simulink model "SingleMerging"  (R2018b)
settings: Solver=VariableStepAuto  StartTime=0.0  StopTime=30  FixedStep=0.1  RelTol=1e-3
PreLoadFcn:
  | init_func
values from neighbouring files (symbols this model uses):
  m = 1650    [CBF_Control.m]    (also in acc.m)
settings Model: Creator=nebneBgnahZ  LastModifiedBy=admin
settings SFSimCC: SimUseLocalCustomCode=off
settings RTWCC: RTWUseLocalCustomCode=off
settings CodeAppCC: StateflowObjectComments=on

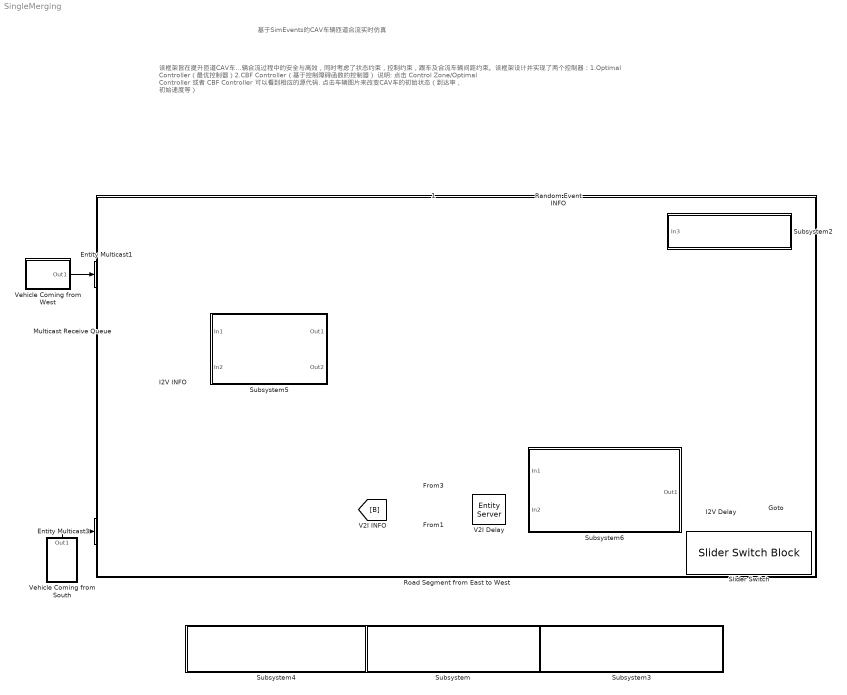
== system SingleMerging ==
  note: 该框架旨在提升匝道CAV车辆合流过程中的安全与高效，同时考虑了状态约束，控制约束，跟车及合流车辆间距约束。该框架设计并实现了两个控制器：1.Optimal Controller（最优控制器）2.CBF Controller（基于控制障碍函数的控制器）
      | 说明:
      | 点击 Control Zone/Optimal Controller 或者 CBF Controller 可以看到相应的源代码.
      | 点击车辆图片来改变CAV车的初始状态（到达率， 初始速度等）
  note: 基于SimEvents的CAV车辆匝道合流实时仿真
  " 1" : Subsystem  mask(Random events){Parameter1=Red Light Violation Warning}
      mask help: Random events do not only refer to vehicle arrival, lane change, and turn, but they also include events that may cause safety issues. Generally, all such random events can be categorized into two classes, depending on whether they are caused by vehicles or by the infrastructure/environment.
      mask TypeOptions Parameter1: Red Light Violation Warning | Curve Speed Warning | Stop Sign Gap Assist | Spot Weather Impact Warning | Reduced Speed/ Work Zone Warning | Pedestrian in Signalized Crosswalk Warning (Transit) | Emergency Electronic Brake Lights (EEBL) | Forward Collision Warning (FCW) | Intersection Movement Assist (IMA) | Left Turn Assist (LTA) | Blind Spot/ Lane Change Warning (BSW/LCW) | Do Not Pass Warning (DNPW) | Vehicle Turning Right in Front of Bus Warning (Transit)
      mask Display:
      | %image('figs/environment.jpg');
      | disp('Random Events')
  Entity Multicast1 : EntityMulticast  InputPortMessageModes=m  MulticastTag=CAV
  Entity Multicast3 : EntityMulticast  InputPortMessageModes=m  MulticastTag=CAV
  I2V Delay : EntityServer  InputPortMessageModes=m  OutputPortMessageModes=m  Capacity=Inf  ServiceTimeValue=0
  Multicast Receive Queue : EntityQueue  OutputPortMessageModes=m  Capacity=100  EntityArrivalSource=Multicast  MulticastTag=CAV
      settings: OutputPortMap=o5
  Road Segment from East to West : Subsystem
      mask Display: image('figs/mergbkg.png');
  Slider Switch : SliderSwitchBlock  WebBlockId=192  LabelPosition=Hide
      settings: Values={{'OC', 'CBF'}, [1 2]}
  Subsystem : Subsystem
      settings: OpenFcn=edit dynamics.m
      mask Display: disp('OC Vehicle Dynamics');
  Subsystem2 : Subsystem
      mask Display: disp('Merging Point')
  Subsystem3 : Subsystem
      settings: OpenFcn=edit fuel_consumption.m
      mask Display: disp('Fuel Consumption Model');
  Subsystem4 : Subsystem
      settings: OpenFcn=edit acc.m
      mask Display: disp('CBF Vehicle Dynamics');
  Subsystem5 : Subsystem
      mask Display:
      | %image('figs/controller.jpg');
      | disp('Control Zone')
  Subsystem6 : Subsystem
      mask Display:
      | %image('figs/coordinator.jpg');
      | disp('Coordinator')
  V2I Delay : EntityServer  InputPortMessageModes=m  OutputPortMessageModes=m  Capacity=Inf  ServiceTimeValue=0.1
  Vehicle Coming from South : Subsystem  mask(Connected Automated Vehicles (CAVs)){modelpopup=Basic model, umin=[], umax=[], vmin=[], vmax=[], length=0, cf=0, cr=0, lf=0, lr=0}
      mask prompts: modelpopup "Vehicle Model Selection"; umin "Maximum Deceleration"; umax "Maximum Acceleration"; vmin "Minimum Speed"; vmax "Maximum Speed"; cf "Front Tire Cornering Stiffness"; cr "Rear Tire Cornering Stiffness"; lf "Distance from CoG to Front Axels"; lr "Distance from CoG to Rear Axels"
      mask help: Vehicles, assumed to be CAVs, should possess the ability to communicate with the controller, the coordinator, and other vehicles in the network. CAVs can differ in driver models, for instance, motion dynamics, control mechanism, and fuel consumption dynamics.
      mask TypeOptions modelpopup: Basic model | Kinematic model | Dynamic model | User-defined
      mask Callback modelpopup:
      | % Get the mask parameter values. This is a cell
      | %   array of character vectors.
      | maskStr = get_param(gcb,'modelpopup');
      | 
      | % The pop-up menu is the first mask parameter.
      | %   Check the value selected in the pop-up
      | if strcmp(maskStr(1),'U')
      | 
      | 
      |     % Set the visibility of both parameters on when
      |     %   User-defined is selected in the pop-up.
      | 
      |     set_param(gcb,'MaskVisibilities',{'on';'on';'on';'on';'on';'on';'on';'on';'on';'on';}),
      | 
      | elseif strcmp(maskStr(1),'B')
      | 
      |     % Turn off the visibility of the Value field
      |     %   when User-defined is not selected.
      | 
      |     set_param(gcb,'MaskVisibilities',{'on';'on';'on';'on';'on';'off';'off';'off';'off';'off';}),
      | 
      |     % Set the character vector in the Values field equal to the
      |     % character vector selected in the Gain pop-up menu.
      | 
      |     %maskStr{2}=maskStr{1};
      | 
      | 
      | elseif strcmp(maskStr(1),'K')
      | 
      |     set_param(gcb,'MaskVisibilities',{'on';'on';'on';'on';'on';'on';'off';'off';'off';'off';}),
      | 
      | else
      | 
      |     set_param(gcb,'MaskVisibilities',{'on';'on';'on';'on';'on';'off';'on';'on';'on';'on';}),
      | 
      | end
      mask Display: image('figs/CAV2.png');
  Vehicle Coming from West : Subsystem  mask(Connected Automated Vehicles (CAVs)){modelpopup=Basic model, umin=[], umax=[], vmin=[], vmax=[], length=0, cf=0, cr=0, lf=0, lr=0}
      mask prompts: modelpopup "Vehicle Model Selection"; umin "Maximum Deceleration"; umax "Maximum Acceleration"; vmin "Minimum Speed"; vmax "Maximum Speed"; cf "Front Tire Cornering Stiffness"; cr "Rear Tire Cornering Stiffness"; lf "Distance from CoG to Front Axels"; lr "Distance from CoG to Rear Axels"
      mask help: Vehicles, assumed to be CAVs, should possess the ability to communicate with the controller, the coordinator, and other vehicles in the network. CAVs can differ in driver models, for instance, motion dynamics, control mechanism, and fuel consumption dynamics.
      mask TypeOptions modelpopup: Basic model | Kinematic model | Dynamic model | User-defined
      mask Callback modelpopup:
      | % Get the mask parameter values. This is a cell
      | %   array of character vectors.
      | maskStr = get_param(gcb,'modelpopup');
      | 
      | % The pop-up menu is the first mask parameter.
      | %   Check the value selected in the pop-up
      | if strcmp(maskStr(1),'U')
      | 
      | 
      |     % Set the visibility of both parameters on when
      |     %   User-defined is selected in the pop-up.
      | 
      |     set_param(gcb,'MaskVisibilities',{'on';'on';'on';'on';'on';'on';'on';'on';'on';'on';}),
      | 
      | elseif strcmp(maskStr(1),'B')
      | 
      |     % Turn off the visibility of the Value field
      |     %   when User-defined is not selected.
      | 
      |     set_param(gcb,'MaskVisibilities',{'on';'on';'on';'on';'on';'off';'off';'off';'off';'off';}),
      | 
      |     % Set the character vector in the Values field equal to the
      |     % character vector selected in the Gain pop-up menu.
      | 
      |     %maskStr{2}=maskStr{1};
      | 
      | 
      | elseif strcmp(maskStr(1),'K')
      | 
      |     set_param(gcb,'MaskVisibilities',{'on';'on';'on';'on';'on';'on';'off';'off';'off';'off';}),
      | 
      | else
      | 
      |     set_param(gcb,'MaskVisibilities',{'on';'on';'on';'on';'on';'off';'on';'on';'on';'on';}),
      | 
      | end
      mask Display: image('figs/CAV.png');
  wires:
  Vehicle Coming from South/1(Out1) -> Entity Multicast3/1
  Vehicle Coming from West/1(Out1) -> Entity Multicast1/1
  I2V Delay/1 -> [A]
  [B] -> V2I Delay/1
  " 1"/1(Out1) -> [C]
  Multicast Receive Queue/1 -> Subsystem5/1(In1)
  [A] -> Subsystem5/2(In2)
  Subsystem5/2(Out2) -> [B]
  [C] -> Subsystem6/1(In1)
  Subsystem6/1(Out1) -> I2V Delay/1
  Subsystem5/1(Out1) -> Subsystem2/1(In3)
  V2I Delay/1 -> Subsystem6/2(In2)

== system SingleMerging/ 1 ==
  Random Event : EntityGenerator  OutputPortMessageModes=m  TimeSource=MATLAB action  IntergenerationTimeAction=dt = 1000;  GenerateEntityAtSimulationStart=off  AttributeName=entity  AttributeInitialValue=0  EntityType=Bus object  EntityTypeName=INFO  EntityPriority=100
  Out1 : Outport
  wires:
  Random Event/1 -> Out1/1

== system SingleMerging/Road Segment from East to West ==

== system SingleMerging/Subsystem ==

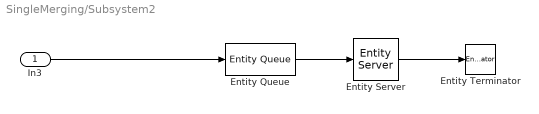
== system SingleMerging/Subsystem2 ==
  In3 : Inport
  Entity Queue : EntityQueue  InputPortMessageModes=m  OutputPortMessageModes=m
      settings: OutputPortMap=o5
  Entity Server : EntityServer  InputPortMessageModes=m  OutputPortMessageModes=m  Capacity=Inf  ServiceTimeSource=MATLAB action  ServiceTimeAction=dt = 30 / entity.FinalSpeed;
  Entity Terminator : EntityTerminator  InputPortMessageModes=m
  wires:
  Entity Queue/1 -> Entity Server/1
  In3/1 -> Entity Queue/1
  Entity Server/1 -> Entity Terminator/1

== system SingleMerging/Subsystem3 ==

== system SingleMerging/Subsystem4 ==

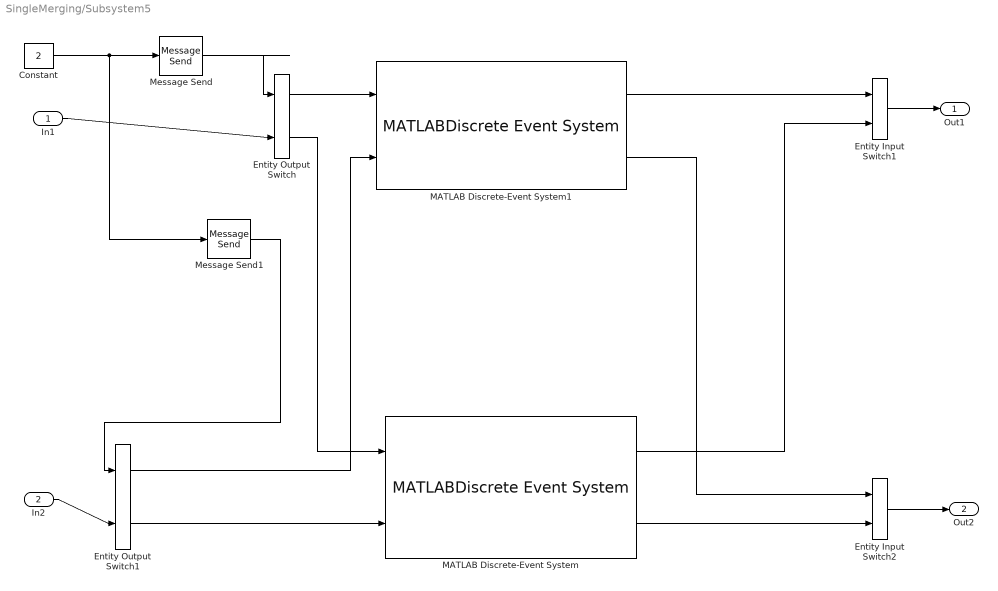
== system SingleMerging/Subsystem5 ==
  In1 : Inport
  In2 : Inport  Port=2
  Constant : Constant  Value=2  SampleTime=-1
  Entity Input Switch1 : EntityInputSwitch  InputPortMessageModes=m,m  OutputPortMessageModes=m  SwitchingCriterion=From control port
  Entity Input Switch2 : EntityInputSwitch  InputPortMessageModes=m,m  OutputPortMessageModes=m  SwitchingCriterion=From control port
  Entity Output Switch : EntityOutputSwitch  InputPortMessageModes=m,m  OutputPortMessageModes=m,m  SwitchingCriterion=From control port  SwitchAttributeName=Attribute1
      settings: InputPortMap=u0,u1
  Entity Output Switch1 : EntityOutputSwitch  InputPortMessageModes=m,m  OutputPortMessageModes=m,m  SwitchingCriterion=From control port  SwitchAttributeName=Attribute1
      settings: InputPortMap=u0,u1
  MATLAB Discrete-Event System : MATLABDiscreteEventSystem  InputPortMessageModes=m,m  OutputPortMessageModes=m,m  System=CBFController  capacity=100  Length=400  step=0.1  Vd=30  Vmax=30  Vmin=0  Umax=0.4  Umin=0.6  SimulateUsing=Interpreted execution
      mask Type: CBFController
      mask Display:
      | disp('CBF Controller');
      | port_label('input',1,'IN');
      | port_label('input',2,'INFO');
      | port_label('output',1,'OUT');
      | port_label('output',2,'INFO');
  MATLAB Discrete-Event System1 : MATLABDiscreteEventSystem  Description=Coordinator  InputPortMessageModes=m,m  OutputPortMessageModes=m,m  System=Controller  capacity=100  step=0.1  L=400  SimulateUsing=Interpreted execution
      mask Type: Controller
      mask Display:
      | disp('OPTIMAL CONTROLLER');
      | port_label('input',1,'IN');
      | port_label('input',2,'INFO');
      | port_label('output',1,'OUT');
      | port_label('output',2,'INFO');
  Message Send : MessageSend  OutputPortMessageModes=m
      settings: InputPortMap=u1
  Message Send1 : MessageSend  OutputPortMessageModes=m
      settings: InputPortMap=u1
  Out1 : Outport
  Out2 : Outport  Port=2
  wires:
  Message Send/1 -> Entity Output Switch/1
  Entity Output Switch1/2 -> MATLAB Discrete-Event System/2
  Entity Output Switch1/1 -> MATLAB Discrete-Event System1/2
  Entity Output Switch/1 -> MATLAB Discrete-Event System1/1
  MATLAB Discrete-Event System/1 -> Entity Input Switch1/2
  MATLAB Discrete-Event System/2 -> Entity Input Switch2/2
  In2/1 -> Entity Output Switch1/2
  Entity Input Switch1/1 -> Out1/1
  Entity Input Switch2/1 -> Out2/1
  Entity Output Switch/2 -> MATLAB Discrete-Event System/1
  MATLAB Discrete-Event System1/2 -> Entity Input Switch2/1
  In1/1 -> Entity Output Switch/2
  Constant/1 -> Message Send/1, Message Send1/1
  MATLAB Discrete-Event System1/1 -> Entity Input Switch1/1
  Message Send1/1 -> Entity Output Switch1/1

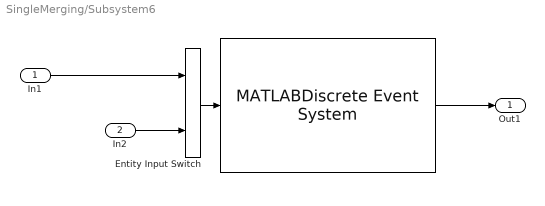
== system SingleMerging/Subsystem6 ==
  In1 : Inport
  In2 : Inport  Port=2
  " " : MATLABDiscreteEventSystem  InputPortMessageModes=m  OutputPortMessageModes=m  System=Coordinator  capacity=100  SimulateUsing=Interpreted execution
      mask Type: Coordinator
      mask Display:
      | disp('COORDINATOR');
      | port_label('input',1,'IN');
      | port_label('output',1,'OUT');
  Entity Input Switch : EntityInputSwitch  InputPortMessageModes=m,m  OutputPortMessageModes=m
  Out1 : Outport
  wires:
  " "/1 -> Out1/1
  In2/1 -> Entity Input Switch/2
  Entity Input Switch/1 -> " "/1
  In1/1 -> Entity Input Switch/1

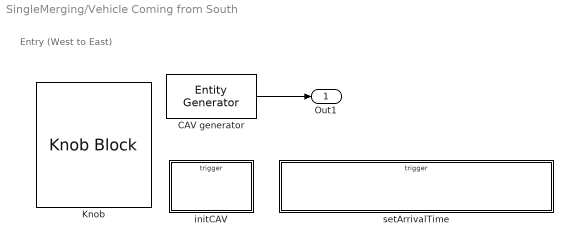
== system SingleMerging/Vehicle Coming from South ==
  note: Entry (West to East)
  "CAV generator " : EntityGenerator  DialogController=slde.AttributeBlockDialog  OutputPortMessageModes=m  TimeSource=MATLAB action  IntergenerationTimeAction=|  GenerateEntityAtSimulationStart=off  GenerateAction=|  AttributeName=ID|Speed|ArrivalTime|FinalSpeed|FinalTime|Position|Destination|Lane|coe  AttributeInitialValue=0|1|1|1|1|1|1|1|[0 0 0 0]  EntityType=Bus object  EntityTypeName=CAV
      IntergenerationTimeAction=|
      | % dt = 2 * rand();
      | %  dt = initCAV2();
      | mean = 0.8;%orin 2.7
      | dt = 2.8- mean*log(1-rand());
      | %dt = 2.8;
      GenerateAction=|
      | entity.FinalSpeed = 30;
      | entity.distance = 0;
      | [entity.ArrivalTime,...
      |     entity.ID] = setArrivalTime2();
      | %entity.Speed = 9 + 3 * rand();
      | entity.Speed = 20;
      | entity.TravelTime = 0;
      | entity.FuelConsumption = 0;
      | entity.Lane = 2;
      | entity.Position = 0;
      | entity.coe = [0, 0, entity.Speed, ...
      |     -entity.Speed * entity.ArrivalTime];
      | dest = [1, 3, 4];
      | idx = ceil(3 * rand()); 
      | entity.Destination = 3;%dest(idx);
      | % 0: go straight 1 : right turn 2: left turn
  Knob : KnobBlock  WebBlockId=193  ScaleMax=1
  initCAV : Subsystem  TreatAsAtomicUnit=on
  setArrivalTime : Subsystem  TreatAsAtomicUnit=on
  Out1 : Outport
  wires:
  "CAV generator "/1 -> Out1/1

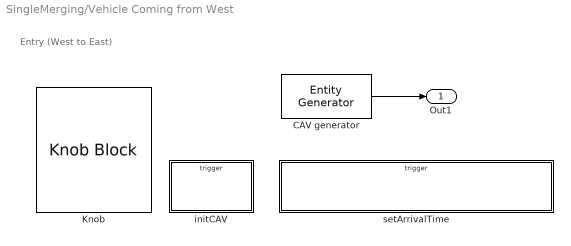
== system SingleMerging/Vehicle Coming from West ==
  note: Entry (West to East)
  "CAV generator " : EntityGenerator  DialogController=slde.AttributeBlockDialog  OutputPortMessageModes=m  TimeSource=MATLAB action  IntergenerationTimeAction=|  GenerateAction=|  AttributeName=ID|Speed|ArrivalTime|FinalSpeed|FinalTime|Position|Lane|Destination|Acceleration|coe  AttributeInitialValue=0|1|1|1|1|0|1|1|1|[0 0 0 0]  EntityType=Bus object  EntityTypeName=CAV
      IntergenerationTimeAction=|
      | % dt = initCAV();
      | mean = 0.2;
      | dt = 1.8 -  mean*log(1-rand());
      | % dt = 2.8;
      | %泊松分布 前面要是不+个数 容易间隔太短
      | % arrive_rate = 0.3;
      | % minTimeInterval = 1.2;
      | % averTimeInterval = 1 / arrive_rate;
      | % maxTimeInterval = averTimeInterval * 1.2;
      | % dt1 = minTimeInterval - log( rand() ) / arrive_rate;
      | % while dt1 > maxTimeInterval
      | %     dt1 = minTimeInterval - log( rand() ) / arrive_rate;
      | % end
      | % dt = dt1;
      GenerateAction=|
      | entity.FinalSpeed = 30;
      | entity.distance = 0;
      | [entity.ArrivalTime,...
      |     entity.ID] = setArrivalTime();
      | %entity.Speed = 8 + 4 * rand();
      | entity.Speed = 20;
      | entity.Lane = 1;
      | entity.Position = 0;
      | entity.TravelTime = 0;
      | entity.FuelConsumption = 0;
      | entity.coe = [0, 0, entity.Speed,...
      |     - entity.Speed * entity.ArrivalTime];
      | dest = [2, 3, 4];
      | idx = ceil(3 * rand()); 
      | entity.Destination = 3;%dest(idx);
      | % 0: go straight 1 : right turn 2: left turn
  Knob : KnobBlock  WebBlockId=194  ScaleMax=3
  initCAV : Subsystem  TreatAsAtomicUnit=on
  setArrivalTime : Subsystem  TreatAsAtomicUnit=on
  Out1 : Outport
  wires:
  "CAV generator "/1 -> Out1/1

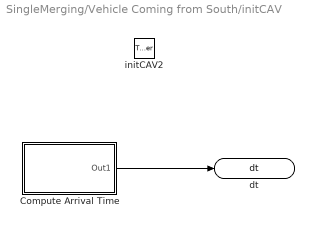
== system SingleMerging/Vehicle Coming from South/initCAV ==
  initCAV2 : TriggerPort  TriggerType=function-call  IsSimulinkFunction=on  FunctionName=initCAV2  FunctionVisibility=scoped  VariantControl=Variant
  "Compute Arrival Time " : Subsystem
  dt : ArgOut  DisableCoverage=on  ArgumentName=dt
  wires:
  "Compute Arrival Time "/1(Out1) -> dt/1

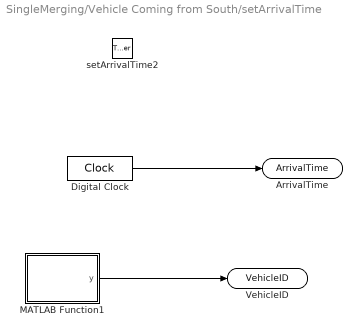
== system SingleMerging/Vehicle Coming from South/setArrivalTime ==
  setArrivalTime2 : TriggerPort  TriggerType=function-call  IsSimulinkFunction=on  FunctionName=setArrivalTime2  FunctionVisibility=scoped  VariantControl=Variant
  Digital Clock : DigitalClock  SampleTime=-1
  MATLAB Function1 : MATLAB Function  TreatAsAtomicUnit=on
  ArrivalTime : ArgOut  DisableCoverage=on  ArgumentName=ArrivalTime
  VehicleID : ArgOut  DisableCoverage=on  Port=2  ArgumentName=VehicleID
  wires:
  Digital Clock/1 -> ArrivalTime/1
  MATLAB Function1/1(y) -> VehicleID/1

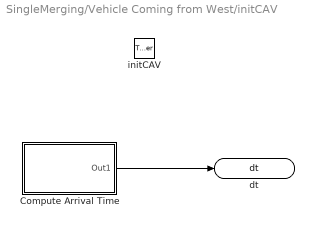
== system SingleMerging/Vehicle Coming from West/initCAV ==
  initCAV : TriggerPort  TriggerType=function-call  IsSimulinkFunction=on  FunctionName=initCAV  FunctionVisibility=scoped  VariantControl=Variant
  "Compute Arrival Time " : Subsystem
  dt : ArgOut  DisableCoverage=on  ArgumentName=dt
  wires:
  "Compute Arrival Time "/1(Out1) -> dt/1

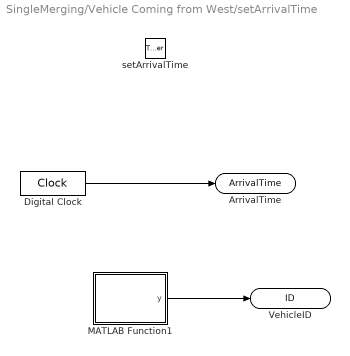
== system SingleMerging/Vehicle Coming from West/setArrivalTime ==
  setArrivalTime : TriggerPort  TriggerType=function-call  IsSimulinkFunction=on  FunctionName=setArrivalTime  FunctionVisibility=scoped  VariantControl=Variant
  Digital Clock : DigitalClock  SampleTime=-1
  MATLAB Function1 : MATLAB Function  TreatAsAtomicUnit=on
  ArrivalTime : ArgOut  DisableCoverage=on  ArgumentName=ArrivalTime
  VehicleID : ArgOut  DisableCoverage=on  Port=2  ArgumentName=ID
  wires:
  Digital Clock/1 -> ArrivalTime/1
  MATLAB Function1/1(y) -> VehicleID/1

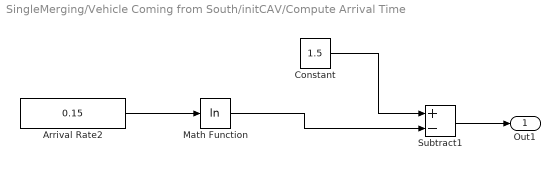
== system SingleMerging/Vehicle Coming from South/initCAV/Compute Arrival Time  ==
  "Arrival Rate2 " : Constant  Value=0.15  SampleTime=-1
  Constant : Constant  Value=1.5  SampleTime=Inf
  Math Function : Math  Operator=log  SaturateOnIntegerOverflow=on
  Subtract1 : Sum  Inputs=+-
  Out1 : Outport
  wires:
  Subtract1/1 -> Out1/1
  Math Function/1 -> Subtract1/2
  Constant/1 -> Subtract1/1
  "Arrival Rate2 "/1 -> Math Function/1

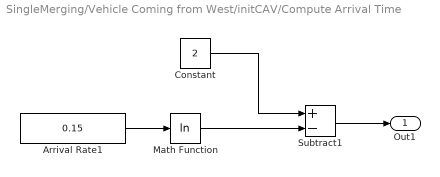
== system SingleMerging/Vehicle Coming from West/initCAV/Compute Arrival Time  ==
  "Arrival Rate1 " : Constant  Value=0.15  SampleTime=-1
  Constant : Constant  Value=2  SampleTime=Inf
  Math Function : Math  Operator=log  SaturateOnIntegerOverflow=on
  Subtract1 : Sum  Inputs=+-
  Out1 : Outport
  wires:
  Subtract1/1 -> Out1/1
  Math Function/1 -> Subtract1/2
  Constant/1 -> Subtract1/1
  "Arrival Rate1 "/1 -> Math Function/1

== matlab function SingleMerging/Vehicle Coming from South/setArrivalTime/MATLAB Function1 ==
  data: y output; FF data_store_memory
function y = getID
global FF

FF = FF + 1;
y = FF;

== matlab function SingleMerging/Vehicle Coming from West/setArrivalTime/MATLAB Function1 ==
  data: y output; FF data_store_memory
function y = getID()
global FF

FF = FF + 1;
y = FF;
